simulink model "problem5"  (R2020b)
settings: Solver=VariableStepAuto  StartTime=0.0  StopTime=10.0  RelTol=1e-3
undefined symbols (not defined in the file): C, R
settings Model: Creator=admin  LastModifiedBy=admin
settings DataIOCC: LoadExternalInput=on  SaveFormat=Array

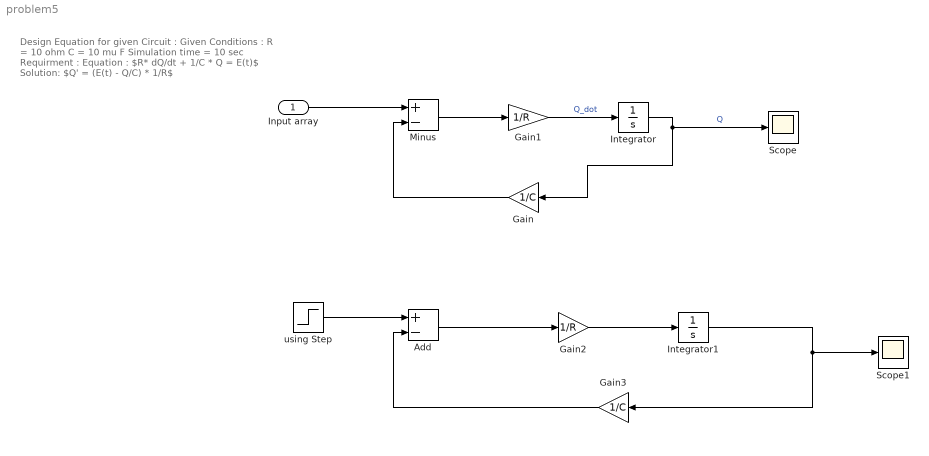
== system problem5 ==
  note: Design Equation for given Circuit :
      |
      | Given Conditions :
      | R = 10 ohm
      | C = 10 mu F
      | Simulation time = 10 sec
      |
      | Requirment :
      | Equation :
      | $R* dQ/dt + 1/C * Q = E(t)$
      |
      | Solution:
      | $Q' = (E(t) - Q/C) * 1/R$
  Input array : Inport
  Add : Sum  Inputs=+-
  Gain : Gain  Gain=1/C
  Gain1 : Gain  Gain=1/R
  Gain2 : Gain  Gain=1/R
  Gain3 : Gain  Gain=1/C
  Integrator : Integrator
  Integrator1 : Integrator
  Minus : Sum  Inputs=+-
  Scope : Scope
  Scope1 : Scope
  using Step : Step  Time=4  Before=2  SampleTime=0
  wires:
  Input array/1 -> Minus/1
  Minus/1 -> Gain1/1
  Gain1/1 -> Integrator/1  "Q_dot"
  Integrator/1 -> Gain/1, Scope/1  "Q"
  Gain/1 -> Minus/2
  using Step/1 -> Add/1
  Gain2/1 -> Integrator1/1
  Gain3/1 -> Add/2
  Add/1 -> Gain2/1
  Integrator1/1 -> Scope1/1, Gain3/1
